simulink model "bai1"  (R2017b)
settings: Solver=ode5  StartTime=0.0  StopTime=2.0  FixedStep=0.001  RelTol=1e-3
libraries: fuzblock x1
settings Model: Creator=phamt  LastModifiedBy=phamt

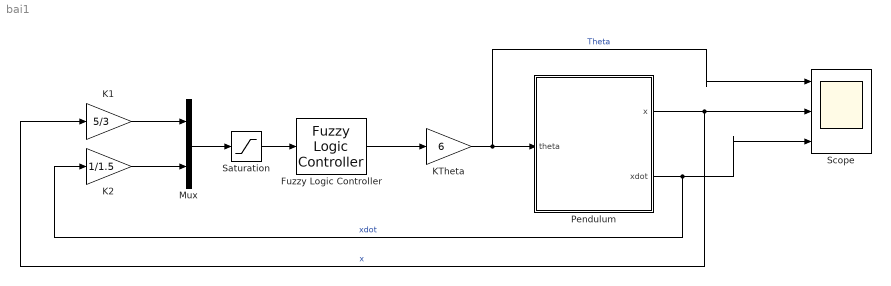
== system bai1 ==
  Fuzzy Logic Controller : fuzblock/Fuzzy Logic  Controller  FIS='bai1_FIS.fis'  OutputSampleNumber=101  DataType=double  FuzzifiedInputs=off  RuleFiringStrengths=off  RuleOutputs=off  AggregatedOutputs=off  SimulateUsing=Interpreted execution
  K1 : Gain  Gain=5/3
  K2 : Gain  Gain=1/1.5
  KTheta : Gain  Gain=6
  Mux : Mux  Inputs=2
  Pendulum : Subsystem  mask{m=0.1, J=0.00005, R=0.02, b=0.01, g=9.81, x0=0.25, xdot0=0}
      mask prompts: m "Khoi luong qua bong"; J "Moment quan tinh cua bong"; R "Ban kinh bong"; b "He so ma sat"; g "Gia toc trong truong"; x0 "Vi tri ban dau"; xdot0 "Van toc ban dau"
  Saturation : Saturate  UpperLimit=1  LowerLimit=-1
  Scope : Scope  NumInputPorts=3
  wires:
  Fuzzy Logic Controller/1 -> KTheta/1
  K1/1 -> Mux/1
  Mux/1 -> Saturation/1
  K2/1 -> Mux/2
  Saturation/1 -> Fuzzy Logic Controller/1
  Pendulum/2(xdot) -> Scope/3, K2/1  "xdot"
  Pendulum/1(x) -> K1/1, Scope/2  "x"
  KTheta/1 -> Scope/1, Pendulum/1(theta)  "Theta"

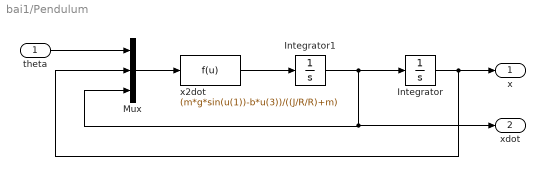
== system bai1/Pendulum ==
  theta : Inport
  Integrator : Integrator  InitialCondition=x0
  Integrator1 : Integrator  InitialCondition=xdot0
  Mux : Mux  Inputs=3
  x2dot : Fcn  Expr=(m*g*sin(u(1))-b*u(3))/((J/R/R)+m)
  x : Outport
  xdot : Outport  Port=2
  wires:
  x2dot/1 -> Integrator1/1
  theta/1 -> Mux/1
  Integrator/1 -> Mux/2, x/1
  Integrator1/1 -> Mux/3, xdot/1, Integrator/1
  Mux/1 -> x2dot/1
